simulink model "cascade_buck_simulink"  (R2026a)
settings: Solver=ode45  StopTime=0.10
undefined symbols (not defined in the file or in its folder): DiscIntNeverNeededParam
settings Model: Creator=hites  LastModifiedBy=hites

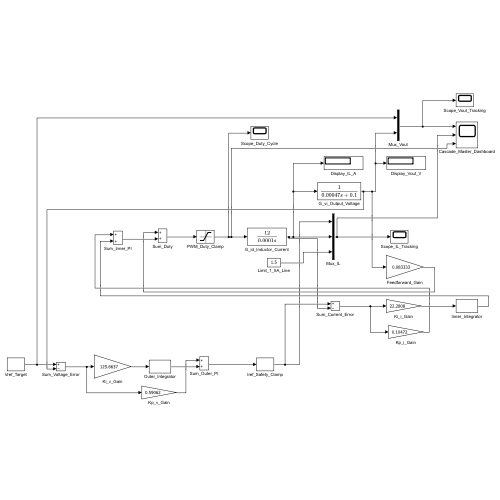
[thumbnail: Simulink's stored preview of the top-level diagram]
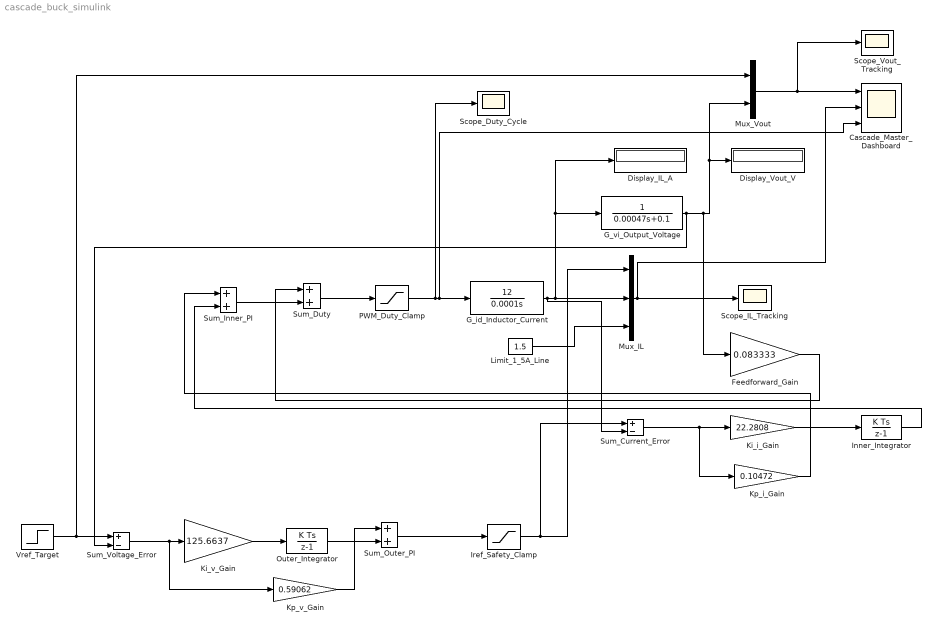
== system cascade_buck_simulink ==
  Cascade_Master_Dashboard : Scope  NumInputPorts=3
  Display_IL_A : Display
  Display_Vout_V : Display
  Feedforward_Gain : Gain  Gain=0.083333
  G_id_Inductor_Current : TransferFcn  Numerator=[12]  Denominator=[0.0001 0]
  G_vi_Output_Voltage : TransferFcn  Denominator=[0.00047 0.1]
  Inner_Integrator : DiscreteIntegrator  SampleTime=0.0001  LimitOutput=on  UpperSaturationLimit=1.0  LowerSaturationLimit=-1.0  ICPrevOutput=DiscIntNeverNeededParam  ICPrevScaledInput=DiscIntNeverNeededParam
  Iref_Safety_Clamp : Saturate  UpperLimit=1.5  LowerLimit=0
  Ki_i_Gain : Gain  Gain=22.2808
  Ki_v_Gain : Gain  Gain=125.6637
  Kp_i_Gain : Gain  Gain=0.10472
  Kp_v_Gain : Gain  Gain=0.59062
  Limit_1_5A_Line : Constant  Value=1.5
  Mux_IL : Mux  Inputs=3
  Mux_Vout : Mux  Inputs=2
  Outer_Integrator : DiscreteIntegrator  SampleTime=0.001  LimitOutput=on  UpperSaturationLimit=1.5  LowerSaturationLimit=0  ICPrevOutput=DiscIntNeverNeededParam  ICPrevScaledInput=DiscIntNeverNeededParam
  PWM_Duty_Clamp : Saturate  UpperLimit=0.9  LowerLimit=0.02
  Scope_Duty_Cycle : Scope
  Scope_IL_Tracking : Scope
  Scope_Vout_Tracking : Scope
  Sum_Current_Error : Sum  Inputs=+-
  Sum_Duty : Sum
  Sum_Inner_PI : Sum
  Sum_Outer_PI : Sum
  Sum_Voltage_Error : Sum  Inputs=+-
  Vref_Target : Step  Time=0  FinalValue=5  SampleTime=0
  wires:
  Sum_Voltage_Error/1 -> Kp_v_Gain/1, Ki_v_Gain/1
  Vref_Target/1 -> Mux_Vout/1, Sum_Voltage_Error/1
  Kp_v_Gain/1 -> Sum_Outer_PI/1
  Sum_Duty/1 -> PWM_Duty_Clamp/1
  Sum_Inner_PI/1 -> Sum_Duty/2
  Ki_v_Gain/1 -> Outer_Integrator/1
  PWM_Duty_Clamp/1 -> Cascade_Master_Dashboard/3, G_id_Inductor_Current/1, Scope_Duty_Cycle/1
  Outer_Integrator/1 -> Sum_Outer_PI/2
  Sum_Outer_PI/1 -> Iref_Safety_Clamp/1
  G_id_Inductor_Current/1 -> G_vi_Output_Voltage/1, Display_IL_A/1, Mux_IL/2, Sum_Current_Error/2
  Limit_1_5A_Line/1 -> Mux_IL/3
  Iref_Safety_Clamp/1 -> Sum_Current_Error/1, Mux_IL/1
  G_vi_Output_Voltage/1 -> Mux_Vout/2, Display_Vout_V/1, Feedforward_Gain/1, Sum_Voltage_Error/2
  Mux_IL/1 -> Cascade_Master_Dashboard/2, Scope_IL_Tracking/1
  Sum_Current_Error/1 -> Kp_i_Gain/1, Ki_i_Gain/1
  Mux_Vout/1 -> Scope_Vout_Tracking/1, Cascade_Master_Dashboard/1
  Feedforward_Gain/1 -> Sum_Duty/1
  Ki_i_Gain/1 -> Inner_Integrator/1
  Kp_i_Gain/1 -> Sum_Inner_PI/1
  Inner_Integrator/1 -> Sum_Inner_PI/2
